simulink model "ejercicio1c"  (R2015b)
settings: Solver=VariableStepAuto  StartTime=0.0  StopTime=1  RelTol=1e-3
libraries: fl_lib x19, nesl_utility x8
settings Model: Creator=xmax1946  LastModifiedBy=xmax1946

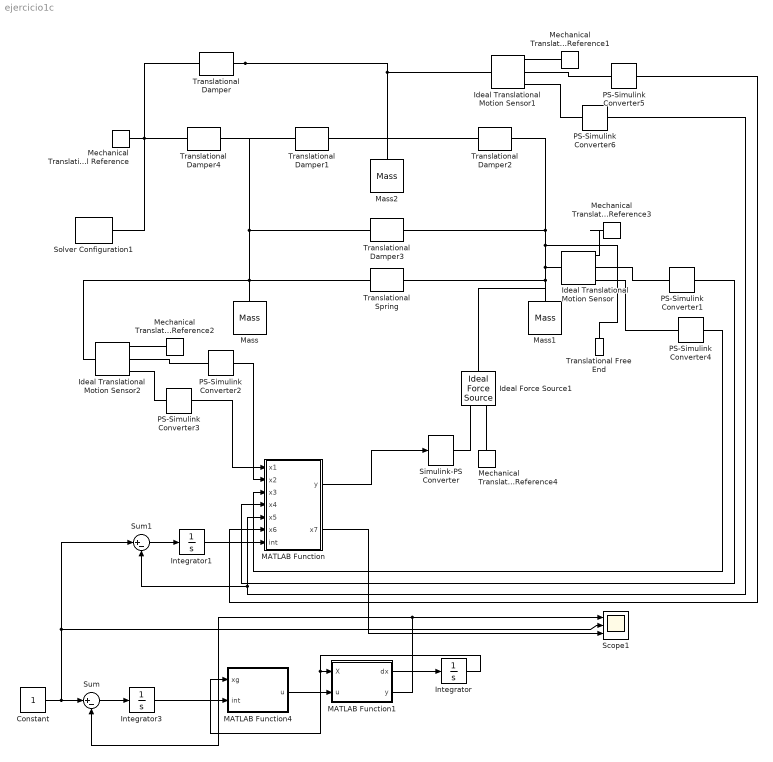
== system ejercicio1c ==
  Constant : Constant
  Ideal Force Source1 : fl_lib/Mechanical/Mechanical Sources/Ideal Force Source
  Ideal Translational Motion Sensor : fl_lib/Mechanical/Mechanical Sensors/Ideal Translational Motion Sensor  offset=0 m
  Ideal Translational Motion Sensor1 : fl_lib/Mechanical/Mechanical Sensors/Ideal Translational Motion Sensor  offset=0 m
  Ideal Translational Motion Sensor2 : fl_lib/Mechanical/Mechanical Sensors/Ideal Translational Motion Sensor  offset=0 m
  Integrator : Integrator  InitialCondition=[0;0;0;0;0;0]  IgnoreLimit=on
  Integrator1 : Integrator  IgnoreLimit=on
  Integrator3 : Integrator  IgnoreLimit=on
  MATLAB Function : MATLAB Function  TreatAsAtomicUnit=on
  MATLAB Function1 : MATLAB Function  TreatAsAtomicUnit=on
  MATLAB Function4 : MATLAB Function  TreatAsAtomicUnit=on
  Mass : fl_lib/Mechanical/Translational Elements/Mass  mass=2 kg  v_specify=off  v_priority=None  v=0 m/s  f_specify=off  f_priority=None  f=0 N
  Mass1 : fl_lib/Mechanical/Translational Elements/Mass  mass=1 kg  v_specify=off  v_priority=None  v=0 m/s  f_specify=off  f_priority=None  f=0 N
  Mass2 : fl_lib/Mechanical/Translational Elements/Mass  mass=1 kg  v_specify=off  v_priority=None  v=0 m/s  f_specify=off  f_priority=None  f=0 N
  Mechanical Translational Reference{,1..4} (5 alike) : fl_lib/Mechanical/Translational Elements/Mechanical Translational Reference
  PS-Simulink Converter{1..6} (6 alike) : nesl_utility/PS-Simulink Converter  PhysicalDomain=network_engine_domain  SubClassName=ps_output  LeftPortType=input  RightPortType=output  PseudoPeriodic=off  Frequencies=[]  Unit=1  AffineConversion=off
  Scope1 : Scope  NumInputPorts=3
  Simulink-PS Converter : nesl_utility/Simulink-PS Converter  PhysicalDomain=network_engine_domain  SubClassName=ps_input  LeftPortType=input  RightPortType=output  PseudoPeriodic=off  Frequencies=[]  NoiseDistribution=none  NoiseParameters=[]  Unit=1  AffineConversion=off  InputFiltering=off  SimscapeFilterOrder=1  InputFilterTimeConstant=0.001  UdotUserProvided=1
  Solver Configuration1 : nesl_utility/Solver Configuration  PhysicalDomain=network_engine_domain  SubClassName=solver  LeftPortType=input  RightPortType=generic  Accelerate=off  Tones=[]  Harmonics=[]  SimulateNoise=off  Profile=off  UseLocalSampling=off  EnableSwitchedLinearOptims=on  FrequencyDomain=off  UseCCode=off  RelTol=0.001  AbsTol=1e-06  MinStep=1e-09  ToWorkspace=off  RevertToSquareIcSolve=off  NumHomotopyIterations=100  PhasorMode=off  PhasorModeNumHarmonics=1  DoDC=off  ResidualTolerance=1e-09  UseLocalSolver=off  LocalSolverChoice=NE_BACKWARD_EULER_ADVANCER  LocalSolverSampleTime=0.001  DoFixedCost=off  MaxNonlinIter=3  MaxModeIter=2  LinearAlgebra=Sparse  DelaysMemoryBudget=1024  AutomaticFiltering=on  FilteringTimeConstant=0.001
  Sum : Sum  Inputs=|+-
  Sum1 : Sum  Inputs=|+-
  Translational Damper{,1..4} (5 alike) : fl_lib/Mechanical/Translational Elements/Translational Damper  D=1 N/(m/s)  v_specify=off  v_priority=None  v=0 m/s  f_specify=off  f_priority=None  f=0 N
  Translational Free End : fl_lib/Mechanical/Translational Elements/Translational Free End  v_specify=off  v_priority=None  v=0 m/s
  Translational Spring : fl_lib/Mechanical/Translational Elements/Translational Spring  spr_rate=2 N/m  v_specify=off  v_priority=None  v=0 m/s  f_specify=off  f_priority=None  f=0 N  x_specify=off  x_priority=None  x=0 m
  wires:
  MATLAB Function1/1(dx) -> Integrator/1
  Integrator/1 -> MATLAB Function4/1(xg), MATLAB Function1/1(X)
  MATLAB Function1/2(y) -> Sum/2, Scope1/1
  Sum/1 -> Integrator3/1
  Integrator3/1 -> MATLAB Function4/2(int)
  MATLAB Function4/1(u) -> MATLAB Function1/2(u)
  PS-Simulink Converter3/1 -> MATLAB Function/1(x1)
  PS-Simulink Converter2/1 -> MATLAB Function/2(x2)
  PS-Simulink Converter4/1 -> MATLAB Function/3(x3)
  PS-Simulink Converter1/1 -> MATLAB Function/4(x4)
  PS-Simulink Converter6/1 -> Sum1/2, MATLAB Function/5(x5)
  PS-Simulink Converter5/1 -> MATLAB Function/6(x6)
  Sum1/1 -> Integrator1/1
  Constant/1 -> Sum1/1, Scope1/2, Sum/1
  Integrator1/1 -> MATLAB Function/7(int)
  MATLAB Function/1(y) -> Simulink-PS Converter/1
  MATLAB Function/2(x7) -> Scope1/3
  connections:
  Solver Configuration1/RConn1 -- Translational Damper4/LConn1 -- Translational Damper/LConn1 -- Mechanical Translational Reference/LConn1
  Translational Spring/LConn1 -- Ideal Translational Motion Sensor2/LConn1 -- Mass/LConn1 -- Translational Damper4/RConn1 -- Translational Damper1/LConn1 -- Translational Damper3/LConn1
  Translational Damper/RConn1 -- Ideal Translational Motion Sensor1/LConn1 -- Mass2/LConn1 -- Translational Damper2/LConn1 -- Translational Damper1/RConn1
  Translational Free End/LConn1 -- Translational Damper2/RConn1 -- Translational Damper3/RConn1 -- Ideal Translational Motion Sensor/LConn1 -- Translational Spring/RConn1 -- Mass1/LConn1 -- Ideal Force Source1/LConn1
  Ideal Translational Motion Sensor/RConn2 -- PS-Simulink Converter1/LConn1
  Mechanical Translational Reference1/LConn1 -- Ideal Translational Motion Sensor1/RConn1
  Mechanical Translational Reference4/LConn1 -- Ideal Force Source1/RConn2
  Mechanical Translational Reference3/LConn1 -- Ideal Translational Motion Sensor/RConn1
  Mechanical Translational Reference2/LConn1 -- Ideal Translational Motion Sensor2/RConn1
  Simulink-PS Converter/RConn1 -- Ideal Force Source1/RConn1
  PS-Simulink Converter2/LConn1 -- Ideal Translational Motion Sensor2/RConn2
  PS-Simulink Converter3/LConn1 -- Ideal Translational Motion Sensor2/RConn3
  PS-Simulink Converter4/LConn1 -- Ideal Translational Motion Sensor/RConn3
  PS-Simulink Converter5/LConn1 -- Ideal Translational Motion Sensor1/RConn2
  PS-Simulink Converter6/LConn1 -- Ideal Translational Motion Sensor1/RConn3

== matlab function ejercicio1c/MATLAB Function1 ==
  data: dx output; X input; y output; u input
function [dx,y]=fcn(X,u)

m1=2;
m2=1;
m3=1;
v1=1;
v2=1;
v3=1;
v4=1;
v5=1;
k=2;
A=[0,1,0,0,0,0;
  -k/m1,(-v2-v4-v1)/m1,k/m1,v2/m1,0,v4/m1
  0,0,0,1,0,0 
  k/m2,v2/m2,-k/m2,(-v2-v5)/m2,0,v5/m2
  0,0,0,0,0,1
  0,v4/m3,0,v5/m3,0,(-v4-v3-v5)/m3
    ];
B=[0;0;0;1/m2;0;0];
C=[0,0,0,0,1,0];

dx=A*X+B*u;
y=C*X;

== matlab function ejercicio1c/MATLAB Function ==
  data: x1 input; y output; x2 input; x3 input; x4 input; x5 input; x6 input; int input; x7 output
function [y,x7] = fcn(x1,x2,x3,x4,x5,x6,int)
kki=2.7056e+06;
kk=[-.81459,.000267,-.8145,.0002665,2.725,.83413]*1e+06;
X=[x1;x2;x3;x4;x5;x6];
x7=x5;
y =int*kki-kk*X;

== matlab function ejercicio1c/MATLAB Function4 ==
  data: xg input; u output; int input
function u = fcn(xg,int)
ki=2.7056e+06;
k=[-.81459,.000267,-.8145,.0002665,2.725,.83413]*1e+06;
u=int*ki-k*xg;
